simulink model "calibModel"  (R2020b)
settings: Solver=FixedStepDiscrete  StartTime=0.0  StopTime=Tf  FixedStep=Ts  RelTol=1e-3  EnableMultiTasking=on
settings Model: PauseTimes=90  PacingRate=3  OrderedModelArguments=off  Creator=sl  LastModifiedBy=sl
settings SolverCC: AutoInsertRateTranBlk=on
settings OptimizationCC: DefaultParameterBehavior=Inlined  EnhancedBackFolding=on  PassReuseOutputArgsAs=Individual arguments  ZeroExternalMemoryAtStartup=off  ZeroInternalMemoryAtStartup=off  MaxStackSize=64  OptimizeBlockOrder=speed  DifferentSizesBufferReuse=on  OptimizationCustomize=off  EfficientTunableParamExpr=on
settings DebuggingCC: ParameterTunabilityLossMsg=error
settings HardwareCC: ProdBitPerPointer=32  ProdBitPerSizeT=32  ProdBitPerPtrDiffT=32  ProdWordSize=32  ProdHWDeviceType=Intel->x86-32 (Windows32)
settings SFSimCC: MATLABDynamicMemAlloc=off
settings RTWCC: Description=Embedded Coder  SystemTargetFile=ert.tlc  GenCodeOnly=on  PackageGeneratedCodeAndArtifacts=on  TemplateMakefile=ert_default_tmf  GenerateReport=on  IncludeHyperlinkInReport=on  LaunchReport=on  GenerateTraceInfo=on  GenerateTraceReport=on  GenerateTraceReportSl=on  GenerateTraceReportSf=on  GenerateTraceReportEml=on
settings CodeAppCC: ForceParamTrailComments=on  IgnoreCustomStorageClasses=off  OperatorAnnotations=on  SimulinkDataObjDesc=on  SFDataObjDesc=on  InsertBlockDesc=on
settings ERTTargetCC: SupportVariableSizeSignals=on  InlinedParameterPlacement=NonHierarchical  ERTCustomFileTemplate=example_file_process.tlc

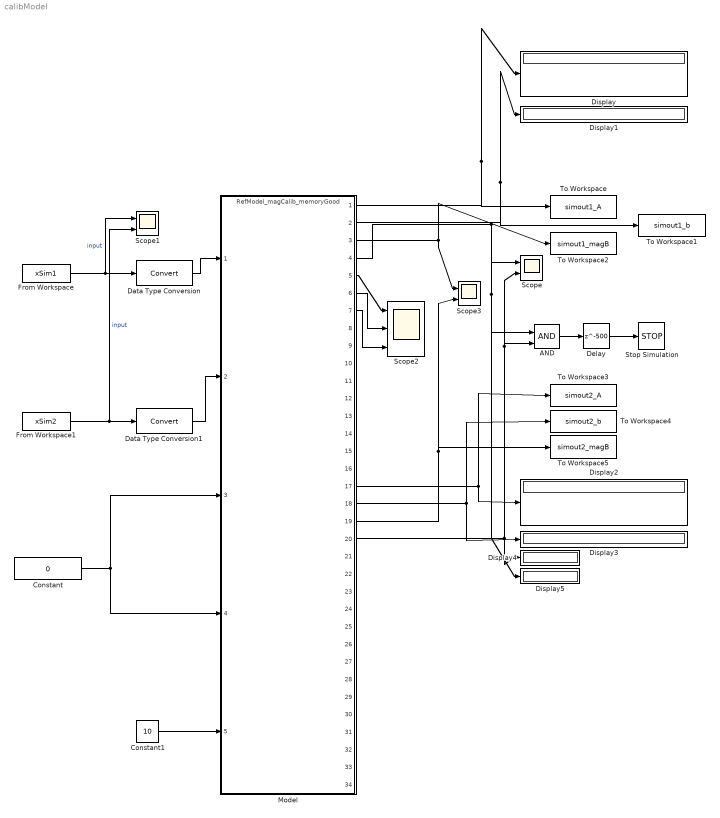
== system calibModel ==
  AND : Logic  IconShape=distinctive  AllPortsSameDT=off  OutDataTypeStr=boolean
  Constant : Constant  Value=0
  Constant1 : Constant  Value=10
  Data Type Conversion : DataTypeConversion
  Data Type Conversion1 : DataTypeConversion
  Delay : Delay  DelayLength=500
  Display{,1..5} (6 alike) : Display
  From Workspace : FromWorkspace  VariableName=xSim1  OutputAfterFinalValue=Holding final value
  From Workspace1 : FromWorkspace  VariableName=xSim2  OutputAfterFinalValue=Holding final value
  Model : ModelReference  ModelNameDialog=RefModel_magCalib_memoryGood.slx  SimulationMode=Normal  ModelReferenceVersion=2.107
  Scope : Scope  NumInputPorts=2
  Scope1 : Scope  NumInputPorts=2
  Scope2 : Scope  NumInputPorts=3
  Scope3 : Scope  NumInputPorts=2
  Stop Simulation : Stop
  To Workspace : ToWorkspace  VariableName=simout1_A  SaveFormat=Timeseries  SampleTime=-1
  To Workspace1 : ToWorkspace  VariableName=simout1_b  SaveFormat=Timeseries  SampleTime=-1
  To Workspace2 : ToWorkspace  VariableName=simout1_magB  SaveFormat=Timeseries  SampleTime=-1
  To Workspace3 : ToWorkspace  VariableName=simout2_A  SaveFormat=Timeseries  SampleTime=-1
  To Workspace4 : ToWorkspace  VariableName=simout2_b  SaveFormat=Timeseries  SampleTime=-1
  To Workspace5 : ToWorkspace  VariableName=simout2_magB  SaveFormat=Timeseries  SampleTime=-1
  wires:
  From Workspace/1 -> Scope1/1, Data Type Conversion/1  "input"
  Model/2 -> To Workspace1/1, Display1/1
  Model/3 -> To Workspace2/1, Scope3/1
  Model/1 -> To Workspace/1, Display/1
  Data Type Conversion/1 -> Model/1
  Model/17 -> Display2/1, To Workspace3/1
  Constant/1 -> Model/4, Model/3
  Model/18 -> Display3/1, To Workspace4/1
  From Workspace1/1 -> Scope1/2, Data Type Conversion1/1  "input"
  Data Type Conversion1/1 -> Model/2
  Model/20 -> Display4/1, AND/2, Scope/2
  Model/4 -> Display5/1, AND/1, Scope/1
  AND/1 -> Delay/1
  Model/7 -> Scope2/3
  Model/6 -> Scope2/2
  Model/5 -> Scope2/1
  Model/19 -> Scope3/2, To Workspace5/1
  Delay/1 -> Stop Simulation/1
  Constant1/1 -> Model/5
